simulink model "sysid_models_v0_2016a"  (R2016a)
settings: Solver=VariableStepAuto  SolverMode=SingleTasking  StartTime=0.0  StopTime=60  RelTol=1e-3
libraries: simulink x1
settings Model: Creator=sprinkle  LastModifiedBy=fangyu
settings DataIOCC: ReturnWorkspaceOutputs=on
settings DebuggingCC: SFUnexpectedBacktrackingDiag=error  SFNoUnconditionalDefaultTransitionDiag=error
settings SFSimCC: SimUseLocalCustomCode=on
settings RTWCC: RTWUseLocalCustomCode=on
settings GRTTargetCC: TargetLangStandard=C99 (ISO)
settings ConfigComp: CovMetricSettings=dwe  CovSaveCumulativeToWorkspaceVar=off  CovSaveSingleToWorkspaceVar=off  CovExternalEMLEnable=on

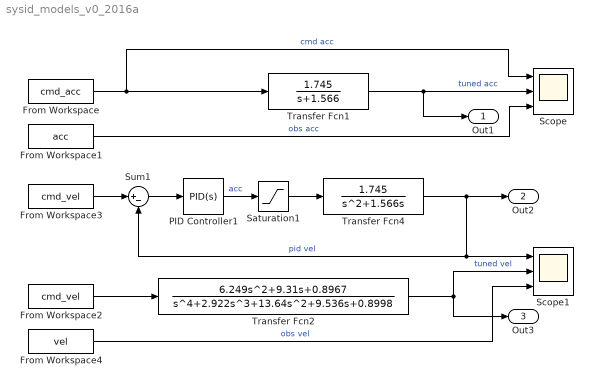
== system sysid_models_v0_2016a ==
  From Workspace : FromWorkspace  VariableName=cmd_acc  SampleTime=0.02
  From Workspace1 : FromWorkspace  VariableName=acc  SampleTime=0.02
  From Workspace2 : FromWorkspace  VariableName=cmd_vel  SampleTime=0.02
  From Workspace3 : FromWorkspace  VariableName=cmd_vel  SampleTime=0.02
  From Workspace4 : FromWorkspace  VariableName=vel  SampleTime=0.02
  PID Controller1 : simulink/Continuous/PID Controller  Controller=PID  Form=Parallel  TimeDomain=Continuous-time  SampleTime=-1  IntegratorMethod=Forward Euler  FilterMethod=Forward Euler  ControllerParametersSource=internal  P=1.0467641274631  I=0.134074922947779  D=1.14032900506104  UseFilter=on  N=2.31488315878784  InitialConditionSource=internal  InitialConditionForIntegrator=0  InitialConditionForFilter=0  DifferentiatorICPrevScaledInput=0  ExternalReset=none  TrackingMode=off  Kt=1  LimitOutput=on  UpperSaturationLimit=1.5  LowerSaturationLimit=-3  LinearizeAsGain=on  AntiWindupMode=clamping  Kb=1  POutMin=[]  POutMax=[]  IOutMin=[]  IOutMax=[]  DOutMin=[]  DOutMax=[]  NOutMin=[]  NOutMax=[]  SumOutMin=[]  SumOutMax=[]  SaturationOutMin=[]  SaturationOutMax=[]  PParamMin=[]  PParamMax=[]  IParamMin=[]  IParamMax=[]  DParamMin=[]  DParamMax=[]  NParamMin=[]  NParamMax=[]  KbParamMin=[]  KbParamMax=[]  KtParamMin=[]  KtParamMax=[]  KbOutMin=[]  KbOutMax=[]  KtOutMin=[]  KtOutMax=[]  IntegratorOutMin=[]  IntegratorOutMax=[]  FilterOutMin=[]  FilterOutMax=[]  SumI1OutMin=[]  SumI1OutMax=[]  SumI2OutMin=[]  SumI2OutMax=[]  SumI3OutMin=[]  SumI3OutMax=[]  SumDOutMin=[]  SumDOutMax=[]  DifferentiatorOutMin=[]  DifferentiatorOutMax=[]  IntegratorContinuousStateAttributes=''  IntegratorStateMustResolveToSignalObject=off  IntegratorRTWStateStorageClass=Auto  FilterContinuousStateAttributes=''  FilterStateMustResolveToSignalObject=off  FilterRTWStateStorageClass=Auto
  Saturation1 : Saturate  UpperLimit=1.5  LowerLimit=-3
  Scope : Scope  NumInputPorts=3
  Scope1 : Scope  NumInputPorts=3
  Sum1 : Sum  Inputs=|+-
  Transfer Fcn1 : TransferFcn  Numerator=[1.745]  Denominator=[1 1.566]
  Transfer Fcn2 : TransferFcn  Numerator=[6.249 9.31 0.8967]  Denominator=[1 2.922 13.64 9.536 0.8998]
  Transfer Fcn4 : TransferFcn  Numerator=[1.745]  Denominator=[1 1.566 0]
  Out1 : Outport
  Out2 : Outport  Port=2
  Out3 : Outport  Port=3
  wires:
  Transfer Fcn1/1 -> Scope/2, Out1/1  "tuned acc"
  From Workspace/1 -> Transfer Fcn1/1, Scope/1  "cmd acc"
  From Workspace1/1 -> Scope/3  "obs acc"
  Transfer Fcn4/1 -> Scope1/1, Sum1/2, Out2/1  "pid vel"
  PID Controller1/1 -> Saturation1/1  "acc"
  Saturation1/1 -> Transfer Fcn4/1
  Sum1/1 -> PID Controller1/1
  From Workspace3/1 -> Sum1/1
  Transfer Fcn2/1 -> Out3/1, Scope1/2  "tuned vel"
  From Workspace2/1 -> Transfer Fcn2/1
  From Workspace4/1 -> Scope1/3  "obs vel"
